simulink model "FLV_simulink"  (R2021b)
settings: Solver=FixedStepAuto  StartTime=0.0  StopTime=10.0  FixedStep=0.01  RelTol=1e-3
values from neighbouring files (symbols this model uses):
  fLenCurve = [ls2, fl_int(:,1)]    [load_data.m]
  fvCurve = [-1 -0.95 -0.9 -0.85 -0.8 -0.75 -0.7 -0.65 -0.6 -0.55 -0.5 -0.45 ... (82 elements, 41x2)]    [force_curves.mat]    (also in load_data.m = [-ls, fv_int])
libraries: simulink x1
settings Model: Creator=rauf  LastModifiedBy=rauf
settings SolverCC: AlgebraicLoopSolver=TrustRegion
settings DebuggingCC: SFMachineParentedDataDiag=warning

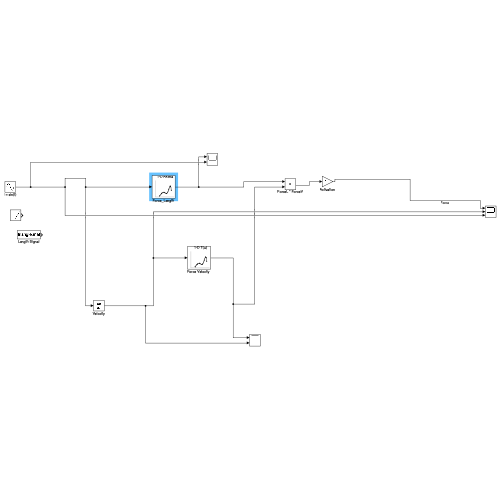
[thumbnail: Simulink's stored preview of the top-level diagram]
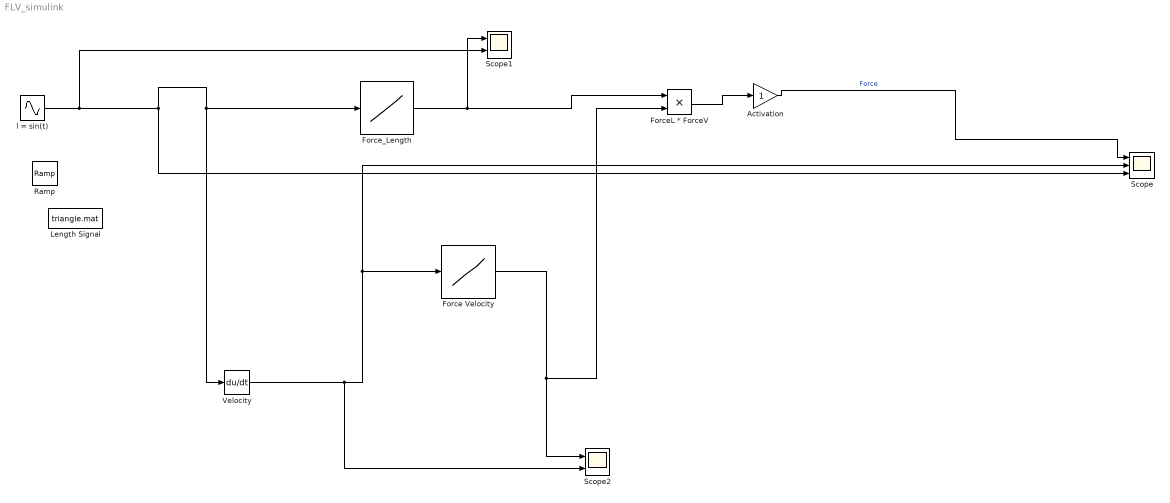
== system FLV_simulink ==
  Activation : Gain
  "Force Velocity " : Lookup_n-D  NumberOfTableDimensions=1  BreakpointsForDimension1=fvCurve(:,1)  Table=fvCurve(:,2)  InterpMethod=Cubic spline  InternalRulePriority=Speed  RndMeth=Simplest  InputSameDT=on
  ForceL * ForceV : Product
  Force_Length : Lookup_n-D  NumberOfTableDimensions=1  BreakpointsForDimension1=fLenCurve(:,1)  Table=fLenCurve(:,2)  InterpMethod=Akima spline  InternalRulePriority=Speed  RndMeth=Simplest  InputSameDT=on
  Length Signal : FromFile  FileName=triangle.mat  SampleTime=0
  Ramp : simulink/Sources/Ramp  slope=1  start=0  InitialOutput=0
  Scope : Scope  NumInputPorts=3
  Scope1 : Scope  NumInputPorts=2
  Scope2 : Scope  NumInputPorts=2
  Velocity : Derivative
  l = sin(t) : Sin  SampleTime=0
  wires:
  l = sin(t)/1 -> Velocity/1, Force_Length/1, Scope/3, Scope1/2
  Velocity/1 -> Scope2/2, "Force Velocity "/1, Scope/2
  Activation/1 -> Scope/1  "Force"
  Force_Length/1 -> ForceL * ForceV/1, Scope1/1
  "Force Velocity "/1 -> Scope2/1, ForceL * ForceV/2
  ForceL * ForceV/1 -> Activation/1
